simulink model "Cansat_Simulation"  (R2026a)
settings: Solver=VariableStepAuto  StopTime=10
libraries: simulink x1
settings Model: Creator=vaish  LastModifiedBy=vaish

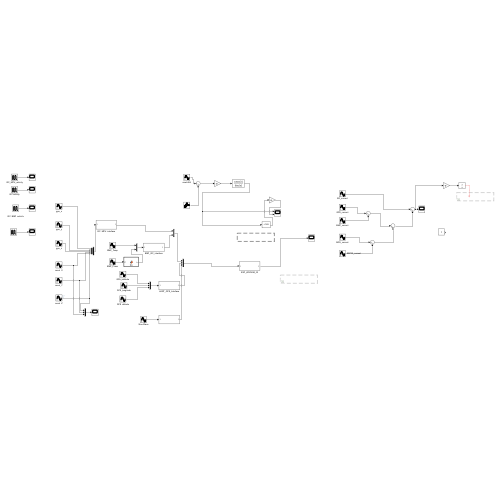
[thumbnail: Simulink's stored preview of the top-level diagram]
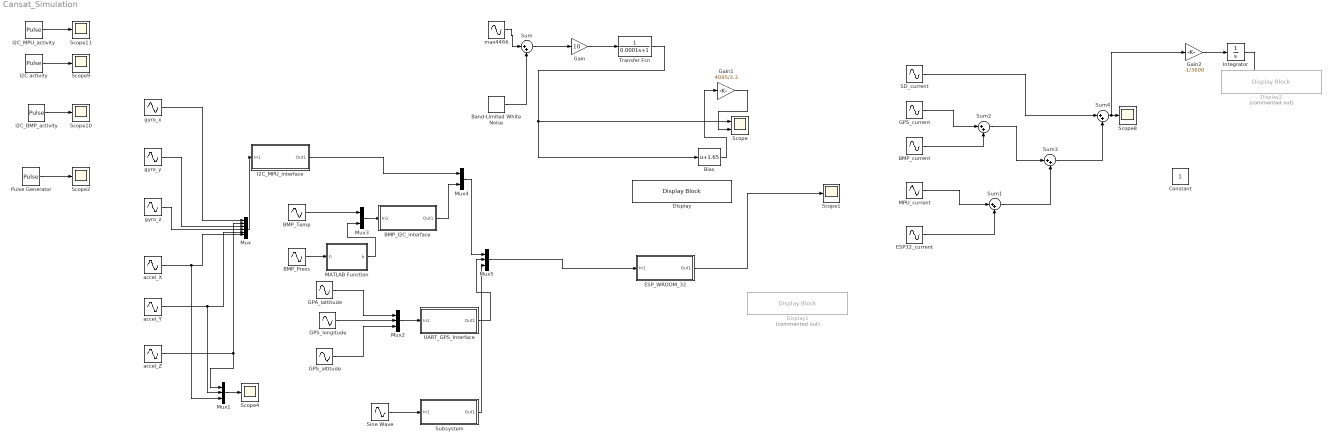
== system Cansat_Simulation ==
  " I2C_BMP_activity" : DiscretePulseGenerator  PulseType=Time based  Period=0.2  PulseWidth=10
  BMP_I2C_interface : Subsystem
  BMP_Press : Sin  Amplitude=2  Bias=1013  Frequency=0.05  SampleTime=0.00001
  BMP_Temp : Sin  Amplitude=5  Bias=25  Frequency=0.1  SampleTime=0.00001
  BMP_current : Sin  Amplitude=0.0005  Bias=0.0007  Frequency=0.2  SampleTime=0.01
  Band-Limited White Noise : simulink/Sources/Band-Limited White Noise  Cov=1e-10  Ts=0.00001  seed=[23341]
  Bias : Bias  Bias=1.65  SaturateOnIntegerOverflow=off
  Constant : Constant
  Display : DisplayBlock  LabelPosition=Hide  Transparency=1  GridColor=[0.502, 0.502, 0.502]
  Display1 : DisplayBlock  Commented=on  LabelPosition=Hide  Transparency=1  GridColor=[0.502, 0.502, 0.502]
  Display2 : DisplayBlock  Commented=on  LabelPosition=Hide  Transparency=1  GridColor=[0.502, 0.502, 0.502]
  ESP32_current : Sin  Amplitude=0.05  Bias=0.08  SampleTime=0.01
  ESP_WROOM_32 : Subsystem
  GPA_lattitude : Sin  Amplitude=0.001  Bias=9.925  Frequency=0.01  SampleTime=0.00001
  GPS_altitude : Sin  Amplitude=2  Bias=100  Frequency=0.005  SampleTime=0.00001
  GPS_current : Sin  Amplitude=0.02  Bias=0.01  Frequency=0.1  SampleTime=0.01
  GPS_longitude : Sin  Amplitude=0.001  Bias=78.119  Frequency=0.008  SampleTime=0.00001
  Gain : Gain  Gain=10
  Gain1 : Gain  Gain=4095/3.3
  Gain2 : Gain  Gain=-1/3600
  I2C activity : DiscretePulseGenerator  PulseType=Time based  Period=0.1  PulseWidth=10
  I2C_MPU_activity : DiscretePulseGenerator  PulseType=Time based  Period=0.2  PulseWidth=10
  I2C_MPU_interface : Subsystem
  Integrator : Integrator  InitialCondition=0.5
  MATLAB Function : MATLAB Function  TreatAsAtomicUnit=on
  MPU_current : Sin  Amplitude=0.002  Bias=0.003  Frequency=0.5  SampleTime=0.01
  Mux : Mux  Inputs=6
  Mux1 : Mux  Inputs=3
  Mux2 : Mux  Inputs=3
  Mux3 : Mux  Inputs=2
  Mux4 : Mux  Inputs=2
  Mux5 : Mux  Inputs=3
  Pulse Generator : DiscretePulseGenerator  PulseType=Time based  Period=0.1  PulseWidth=10
  SD_current : Sin  Amplitude=0.015  Bias=0.025  Frequency=0.3  SampleTime=0.01
  Scope : Scope  NumInputPorts=2
      settings: ActiveDisplayYMinimum=-495.32859866618287  ActiveDisplayYMaximum=3048.6771674828133
  Scope{1..2,4,8..11} (7 alike) : Scope
      Scope1 settings: ActiveDisplayYMinimum=-35.012494792302704  ActiveDisplayYMaximum=115.11245313086027
      Scope10 settings: ActiveDisplayYMinimum=-1  ActiveDisplayYMaximum=1  DataLoggingVariableName=ScopeData10
      Scope11 settings: ActiveDisplayYMinimum=-1  ActiveDisplayYMaximum=1  DataLoggingVariableName=ScopeData11
      Scope2 settings: ActiveDisplayYMinimum=-0.12499999999999997  ActiveDisplayYMaximum=1.125  DataLoggingVariableName=ScopeData2
      Scope4 settings: ActiveDisplayYMinimum=-1  ActiveDisplayYMaximum=1  DataLoggingVariableName=ScopeData4
      Scope8 settings: ActiveDisplayYMinimum=0.040699338112722874  ActiveDisplayYMaximum=0.23198377178466517  DataLoggingVariableName=ScopeData8
      Scope9 settings: ActiveDisplayYMinimum=-1  ActiveDisplayYMaximum=1  DataLoggingVariableName=ScopeData9
  Sine Wave : Sin  Frequency=0.5  SampleTime=0.00001
  Subsystem : Subsystem
  Sum{,1..4} (5 alike) : Sum  Inputs=|++
  Transfer Fcn : TransferFcn  Denominator=[0.0001 1]
  UART_GPS_Interface : Subsystem
  accel_X : Sin  Amplitude=0.2  Frequency=2  SampleTime=0.00001
  accel_Y : Sin  Amplitude=0.1  SampleTime=0.00001
  accel_Z : Sin  Amplitude=0.05  Frequency=0.5  SampleTime=0.00001
  gyro_x : Sin  Amplitude=20  Frequency=6.283  Phase=0.00001  SampleTime=0.00001
  gyro_y : Sin  Amplitude=10  Frequency=3.1416  SampleTime=0.00001
  gyro_z : Sin  Amplitude=5  Bias=1  Frequency=1.2566  SampleTime=0.00001
  max4466 : Sin  Amplitude=0.1  Frequency=20000  SampleTime=0.00001
  wires:
  Transfer Fcn/1 -> Bias/1, Scope/1
  max4466/1 -> Sum/1
  Bias/1 -> Gain1/1
  Gain1/1 -> Scope/2
  Gain/1 -> Transfer Fcn/1
  Sum/1 -> Gain/1
  Band-Limited White Noise/1 -> Sum/2
  BMP_Temp/1 -> Mux3/1
  BMP_Press/1 -> MATLAB Function/1(P)
  MATLAB Function/1(h) -> Mux3/2
  gyro_y/1 -> Mux/3
  gyro_z/1 -> Mux/4
  accel_X/1 -> Mux1/3, Mux/6
  accel_Y/1 -> Mux1/2, Mux/5
  accel_Z/1 -> Mux1/1, Mux/2
  gyro_x/1 -> Mux/1
  Mux/1 -> I2C_MPU_interface/1(In1)
  Mux1/1 -> Scope4/1
  GPA_lattitude/1 -> Mux2/1
  GPS_longitude/1 -> Mux2/2
  Mux2/1 -> UART_GPS_Interface/1(In1)
  I2C activity/1 -> Scope9/1
  " I2C_BMP_activity"/1 -> Scope10/1
  I2C_MPU_activity/1 -> Scope11/1
  Mux3/1 -> BMP_I2C_interface/1(In1)
  I2C_MPU_interface/1(Out1) -> Mux4/1
  Mux4/1 -> Mux5/1
  BMP_I2C_interface/1(Out1) -> Mux4/2
  ESP_WROOM_32/1(Out1) -> Scope1/1
  GPS_altitude/1 -> Mux2/3
  UART_GPS_Interface/1(Out1) -> Mux5/2
  Mux5/1 -> ESP_WROOM_32/1(In1)
  Sine Wave/1 -> Subsystem/1(In1)
  Subsystem/1(Out1) -> Mux5/3
  Pulse Generator/1 -> Scope2/1
  ESP32_current/1 -> Sum1/2
  MPU_current/1 -> Sum1/1
  BMP_current/1 -> Sum2/2
  GPS_current/1 -> Sum2/1
  SD_current/1 -> Sum4/1
  Sum2/1 -> Sum3/1
  Sum1/1 -> Sum3/2
  Sum3/1 -> Sum4/2
  Sum4/1 -> Gain2/1, Scope8/1
  Gain2/1 -> Integrator/1
  Integrator/1 -> ?

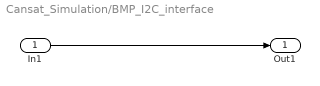
== system Cansat_Simulation/BMP_I2C_interface ==
  In1 : Inport
  Out1 : Outport
  wires:
  In1/1 -> Out1/1

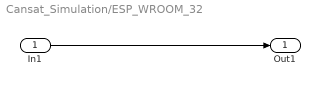
== system Cansat_Simulation/ESP_WROOM_32 ==
  In1 : Inport
  Out1 : Outport
  wires:
  In1/1 -> Out1/1

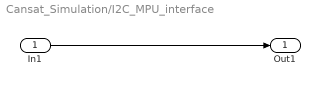
== system Cansat_Simulation/I2C_MPU_interface ==
  In1 : Inport
  Out1 : Outport
  wires:
  In1/1 -> Out1/1
  ? -> ?

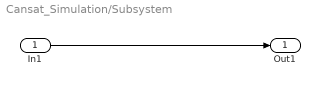
== system Cansat_Simulation/Subsystem ==
  In1 : Inport
  Out1 : Outport
  wires:
  In1/1 -> Out1/1

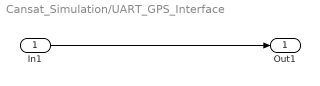
== system Cansat_Simulation/UART_GPS_Interface ==
  In1 : Inport
  Out1 : Outport
  wires:
  In1/1 -> Out1/1

== matlab function Cansat_Simulation/MATLAB Function ==
  data: h output; P input
function h = fcn(P)
h = 44330 * (1 - (P/1013.25)^(1/5.255));
end
